simulink model "Adaptive_Cruise_Control"  (R2019b)
settings: Solver=FixedStepDiscrete  StartTime=0.0  StopTime=10.0  RelTol=1e-3
settings Model: DataDictionary=Adaptive_Cruise_Control_DataDictionary.sldd  EnableAccessToBaseWorkspace=off  Creator=user  LastModifiedBy=user
settings OptimizationCC: DefaultParameterBehavior=Inlined  UseDivisionForNetSlopeComputation=on  GainParamInheritBuiltInType=on  UseFloatMulNetSlope=on  InlineInvariantSignals=on  PassReuseOutputArgsAs=Individual arguments  ZeroExternalMemoryAtStartup=off  ZeroInternalMemoryAtStartup=off  NoFixptDivByZeroProtection=on  EfficientFloat2IntCast=on  LifeSpan=1  OptimizeBlockOrder=speed  DifferentSizesBufferReuse=on  EfficientTunableParamExpr=on
settings DebuggingCC: ParameterTunabilityLossMsg=error
settings HardwareCC: ProdLongLongMode=on
settings SFSimCC: MATLABDynamicMemAlloc=off
settings RTWCC: SystemTargetFile=ert.tlc  TemplateMakefile=ert_default_tmf  GenerateReport=on  IncludeHyperlinkInReport=on  LaunchReport=on  GenerateTraceInfo=on  GenerateTraceReport=on  GenerateTraceReportSl=on  GenerateTraceReportSf=on  GenerateTraceReportEml=on  GenerateCodeMetricsReport=on
settings CodeAppCC: ForceParamTrailComments=on  IgnoreCustomStorageClasses=off  OperatorAnnotations=on  SimulinkDataObjDesc=on  SFDataObjDesc=on  CustomSymbolStrGlobalVar=rt$N$M  CustomSymbolStrType=$N$M  CustomSymbolStrFcn=$N$M$F  CustomSymbolStrMacro=$N$M  InsertBlockDesc=on
settings ERTTargetCC: TargetLangStandard=C99 (ISO)  GenerateSampleERTMain=on  IncludeMdlTerminateFcn=off  CombineSignalStateStructs=on  SupportAbsoluteTime=off  SupportNonFinite=off  SupportComplex=off  SupportNonInlinedSFcns=on  InlinedParameterPlacement=NonHierarchical  ERTCustomFileTemplate=example_file_process.tlc  ERTFilePackagingFormat=CompactWithDataFile

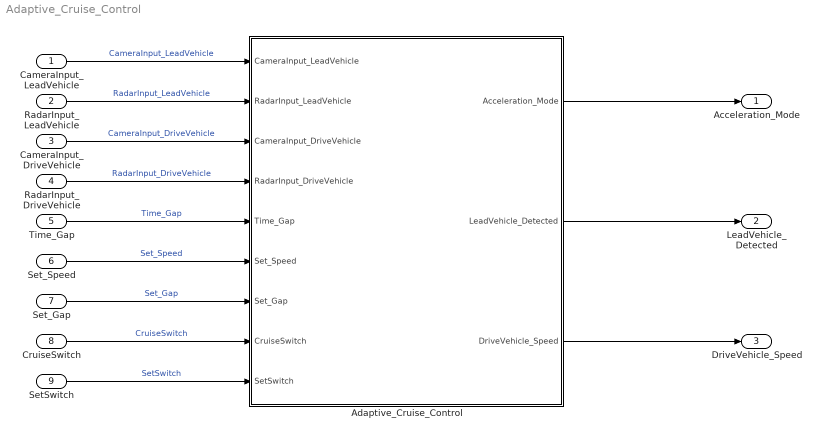
== system Adaptive_Cruise_Control ==
  CameraInput_LeadVehicle : Inport  OutMin=0  OutMax=255  OutDataTypeStr=uint8  PortDimensions=1  SampleTime=0.01
  RadarInput_LeadVehicle : Inport  Port=2  OutMin=0  OutMax=255  OutDataTypeStr=uint8  PortDimensions=1  SampleTime=0.01
  CameraInput_DriveVehicle : Inport  Port=3  OutMin=0  OutMax=255  OutDataTypeStr=uint8  PortDimensions=1  SampleTime=0.01
  RadarInput_DriveVehicle : Inport  Port=4  OutMin=0  OutMax=255  OutDataTypeStr=uint8  PortDimensions=1  SampleTime=0.01
  Time_Gap : Inport  Port=5  OutMin=0  OutMax=255  OutDataTypeStr=uint8  PortDimensions=1  SampleTime=0.01
  Set_Speed : Inport  Port=6  OutMin=0  OutMax=255  OutDataTypeStr=uint8  PortDimensions=1  SampleTime=0.01
  Set_Gap : Inport  Port=7  OutMin=0  OutMax=255  OutDataTypeStr=uint8  PortDimensions=1  SampleTime=0.01
  CruiseSwitch : Inport  Port=8  OutMin=0  OutMax=1  OutDataTypeStr=boolean  PortDimensions=1  SampleTime=0.01
  SetSwitch : Inport  Port=9  OutMin=0  OutMax=1  OutDataTypeStr=boolean  PortDimensions=1  SampleTime=0.01
  Adaptive_Cruise_Control : Subsystem
  Acceleration_Mode : Outport
  LeadVehicle_Detected : Outport  Port=2
  DriveVehicle_Speed : Outport  Port=3
  wires:
  CameraInput_LeadVehicle/1 -> Adaptive_Cruise_Control/1(CameraInput_LeadVehicle)  "CameraInput_LeadVehicle"
  RadarInput_LeadVehicle/1 -> Adaptive_Cruise_Control/2(RadarInput_LeadVehicle)  "RadarInput_LeadVehicle"
  CameraInput_DriveVehicle/1 -> Adaptive_Cruise_Control/3(CameraInput_DriveVehicle)  "CameraInput_DriveVehicle"
  RadarInput_DriveVehicle/1 -> Adaptive_Cruise_Control/4(RadarInput_DriveVehicle)  "RadarInput_DriveVehicle"
  Time_Gap/1 -> Adaptive_Cruise_Control/5(Time_Gap)  "Time_Gap"
  Set_Speed/1 -> Adaptive_Cruise_Control/6(Set_Speed)  "Set_Speed"
  Set_Gap/1 -> Adaptive_Cruise_Control/7(Set_Gap)  "Set_Gap"
  Adaptive_Cruise_Control/1(Acceleration_Mode) -> Acceleration_Mode/1
  Adaptive_Cruise_Control/2(LeadVehicle_Detected) -> LeadVehicle_Detected/1
  Adaptive_Cruise_Control/3(DriveVehicle_Speed) -> DriveVehicle_Speed/1
  CruiseSwitch/1 -> Adaptive_Cruise_Control/8(CruiseSwitch)  "CruiseSwitch"
  SetSwitch/1 -> Adaptive_Cruise_Control/9(SetSwitch)  "SetSwitch"

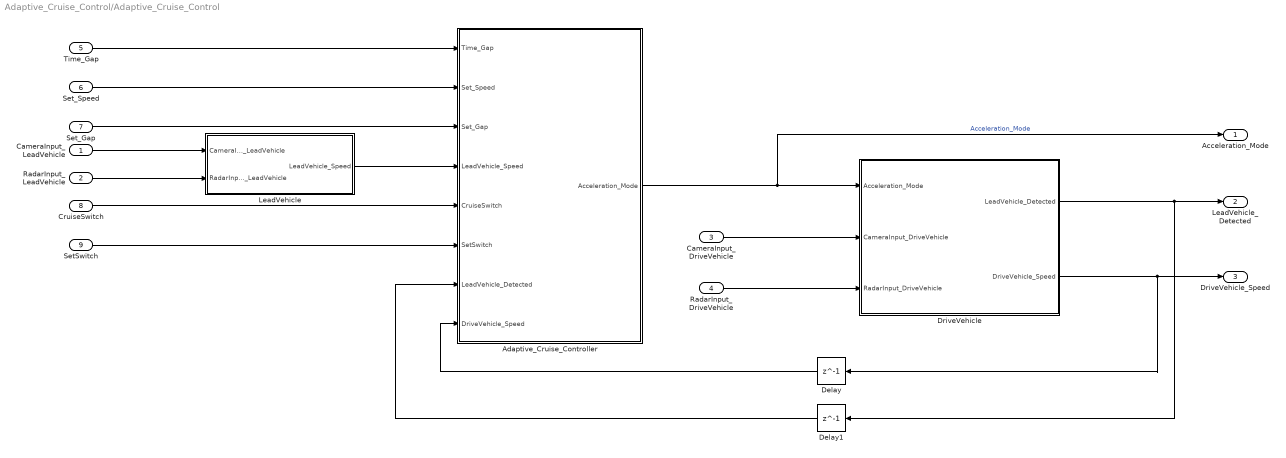
== system Adaptive_Cruise_Control/Adaptive_Cruise_Control ==
  CameraInput_LeadVehicle : Inport
  RadarInput_LeadVehicle : Inport  Port=2
  CameraInput_DriveVehicle : Inport  Port=3
  RadarInput_DriveVehicle : Inport  Port=4
  Time_Gap : Inport  Port=5
  Set_Speed : Inport  Port=6
  Set_Gap : Inport  Port=7
  CruiseSwitch : Inport  Port=8
  SetSwitch : Inport  Port=9
  Adaptive_Cruise_Controller : Stateflow chart  BlockKeywords=__PRM__SERIALIZED__DATA__:Stateflow Chart,Stateflow Diagram  TreatAsAtomicUnit=on
  Delay : Delay  DelayLength=1  SampleTime=0.01
  Delay1 : Delay  DelayLength=1  SampleTime=0.01
  DriveVehicle : Subsystem
  LeadVehicle : Subsystem
  Acceleration_Mode : Outport
  LeadVehicle_Detected : Outport  Port=2
  DriveVehicle_Speed : Outport  Port=3
  wires:
  CameraInput_DriveVehicle/1 -> DriveVehicle/2(CameraInput_DriveVehicle)
  RadarInput_DriveVehicle/1 -> DriveVehicle/3(RadarInput_DriveVehicle)
  RadarInput_LeadVehicle/1 -> LeadVehicle/2(RadarInput_LeadVehicle)
  CameraInput_LeadVehicle/1 -> LeadVehicle/1(CameraInput_LeadVehicle)
  Adaptive_Cruise_Controller/1(Acceleration_Mode) -> DriveVehicle/1(Acceleration_Mode), Acceleration_Mode/1  "Acceleration_Mode"
  DriveVehicle/2(DriveVehicle_Speed) -> DriveVehicle_Speed/1, Delay/1
  Time_Gap/1 -> Adaptive_Cruise_Controller/1(Time_Gap)
  Set_Speed/1 -> Adaptive_Cruise_Controller/2(Set_Speed)
  Set_Gap/1 -> Adaptive_Cruise_Controller/3(Set_Gap)
  LeadVehicle/1(LeadVehicle_Speed) -> Adaptive_Cruise_Controller/4(LeadVehicle_Speed)
  DriveVehicle/1(LeadVehicle_Detected) -> LeadVehicle_Detected/1, Delay1/1
  CruiseSwitch/1 -> Adaptive_Cruise_Controller/5(CruiseSwitch)
  SetSwitch/1 -> Adaptive_Cruise_Controller/6(SetSwitch)
  Delay/1 -> Adaptive_Cruise_Controller/8(DriveVehicle_Speed)
  Delay1/1 -> Adaptive_Cruise_Controller/7(LeadVehicle_Detected)

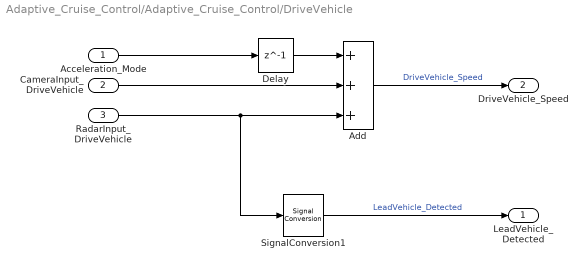
== system Adaptive_Cruise_Control/Adaptive_Cruise_Control/DriveVehicle ==
  Acceleration_Mode : Inport
  CameraInput_DriveVehicle : Inport  Port=2
  RadarInput_DriveVehicle : Inport  Port=3
  Add : Sum  Inputs=+++
  Delay : Delay  DelayLength=1  SampleTime=0.01
  SignalConversion1 : SignalConversion  OverrideOpt=off
  LeadVehicle_Detected : Outport
  DriveVehicle_Speed : Outport  Port=2
  wires:
  Add/1 -> DriveVehicle_Speed/1  "DriveVehicle_Speed"
  Acceleration_Mode/1 -> Delay/1
  CameraInput_DriveVehicle/1 -> Add/2
  RadarInput_DriveVehicle/1 -> Add/3, SignalConversion1/1
  SignalConversion1/1 -> LeadVehicle_Detected/1  "LeadVehicle_Detected"
  Delay/1 -> Add/1

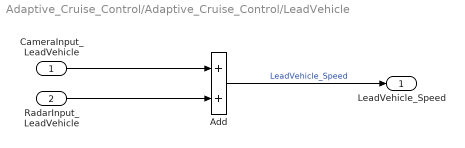
== system Adaptive_Cruise_Control/Adaptive_Cruise_Control/LeadVehicle ==
  CameraInput_LeadVehicle : Inport
  RadarInput_LeadVehicle : Inport  Port=2
  Add : Sum
  LeadVehicle_Speed : Outport
  wires:
  CameraInput_LeadVehicle/1 -> Add/1
  RadarInput_LeadVehicle/1 -> Add/2
  Add/1 -> LeadVehicle_Speed/1  "LeadVehicle_Speed"

== stateflow chart Adaptive_Cruise_Control/Adaptive_Cruise_Controller ==
  state ACC_ACTIVE_MODE
    state LeadVehicle_Not_Detected
      en:
      Acceleration_Mode = 1;
    state LeadVehicle_Speed_lessthan_Set_Speed
      en:
      Acceleration_Mode = 4;
    state LeadVehicle_Detected_Follow
      en:
      Acceleration_Mode = 2;
    state LeadVehicle_Speed_equal_Set_Speed
      en:
      Acceleration_Mode = 5;
    state LeadVehicle_Detected_Resume
      en:
      Acceleration_Mode = 3;
    state LeadVehicle_Not_Detected_Resume
      en:
      Acceleration_Mode = 1;
    LeadVehicle_Not_Detected -> LeadVehicle_Speed_lessthan_Set_Speed [order 2] : [(LeadVehicle_Detected == 1)...
        | && (LeadVehicle_Speed < Set_Speed)...
        | || (Time_Gap < Set_Gap)]
    LeadVehicle_Speed_lessthan_Set_Speed -> LeadVehicle_Not_Detected [order 1] : [(LeadVehicle_Detected == 0) && (DriveVehicle_Speed == Set_Speed)]
    LeadVehicle_Not_Detected -> LeadVehicle_Detected_Follow [order 1] : [(LeadVehicle_Detected==1) && (DriveVehicle_Speed == Set_Speed)...
        | && (LeadVehicle_Speed >= Set_Speed) && (Time_Gap >= Set_Gap)]
    LeadVehicle_Detected_Follow -> LeadVehicle_Not_Detected [order 1] : [LeadVehicle_Detected==0]
    LeadVehicle_Detected_Follow -> LeadVehicle_Speed_lessthan_Set_Speed [order 2] : [(LeadVehicle_Detected == 1) && (LeadVehicle_Speed < Set_Speed) || (Time_Gap < Set_Gap)]
    LeadVehicle_Speed_lessthan_Set_Speed -> LeadVehicle_Speed_equal_Set_Speed [order 2] : [((LeadVehicle_Speed*1.25>=DriveVehicle_Speed)...
        | && (LeadVehicle_Speed * 0.75<=DriveVehicle_Speed))...
        | && (DriveVehicle_Speed < Set_Speed)...
        | && ((Time_Gap<=1.25*Set_Gap)...
        | && (Time_Gap >=0.75*Set_Gap))]
    LeadVehicle_Speed_equal_Set_Speed -> LeadVehicle_Speed_lessthan_Set_Speed [order 3] : [(LeadVehicle_Speed<Set_Speed)...
        | && (LeadVehicle_Speed<DriveVehicle_Speed)...
        | || (Time_Gap==0.75*Set_Gap)]
    (default) -> LeadVehicle_Detected_Follow
    LeadVehicle_Detected_Resume -> LeadVehicle_Detected_Follow [order 1] : [(DriveVehicle_Speed == Set_Speed)...
        | && (LeadVehicle_Speed >= Set_Speed) && (Time_Gap >= Set_Gap)]
    LeadVehicle_Speed_equal_Set_Speed -> LeadVehicle_Detected_Resume [order 2] : [(DriveVehicle_Speed < Set_Speed) && (LeadVehicle_Speed > DriveVehicle_Speed) || (Time_Gap >= Set_Gap)]
    LeadVehicle_Detected_Resume -> LeadVehicle_Speed_equal_Set_Speed [order 3] : [(DriveVehicle_Speed < Set_Speed) && (LeadVehicle_Speed == DriveVehicle_Speed) && (Time_Gap == Set_Gap)]
    LeadVehicle_Speed_equal_Set_Speed -> LeadVehicle_Not_Detected_Resume [order 1] : [(LeadVehicle_Detected == 0) || (DriveVehicle_Speed <= Set_Speed)]
    LeadVehicle_Detected_Resume -> LeadVehicle_Not_Detected_Resume [order 2] : [LeadVehicle_Detected==0]
  state ACC_STANDBY_MODE
    en:
    Acceleration_Mode = 1;
  state ACC_OFF_MODE
    en:
    Acceleration_Mode = 0;
  ACC_ACTIVE_MODE -> ACC_OFF_MODE [order 1] : [CruiseSwitch == 0]
  ACC_STANDBY_MODE -> ACC_ACTIVE_MODE [order 2] : [SetSwitch == 1]
  ACC_ACTIVE_MODE -> ACC_STANDBY_MODE [order 2] : [SetSwitch == 0]
  ACC_OFF_MODE -> ACC_STANDBY_MODE : [CruiseSwitch == 1]
  (default) -> ACC_OFF_MODE
  ACC_STANDBY_MODE -> ACC_OFF_MODE [order 1] : [CruiseSwitch == 0]
  data: Time_Gap input; Set_Speed input; Set_Gap input; LeadVehicle_Speed input; CruiseSwitch input; SetSwitch input; LeadVehicle_Detected input; DriveVehicle_Speed input; Acceleration_Mode output
